simulink model "motor"  (R2015a)
settings: Solver=ode45  StartTime=0.0  StopTime=10.0  RelTol=1e-3
libraries: simulink x2
settings Model: Creator=joselo  LastModifiedBy=joselo

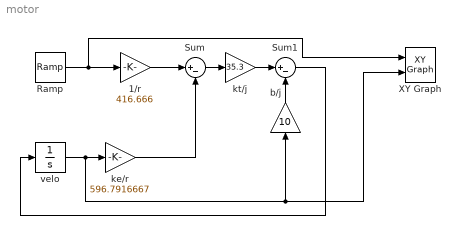
== system motor ==
  1/r : Gain  Gain=416.666
  Ramp : simulink/Sources/Ramp  slope=1  start=0  X0=0
  Sum : Sum  Inputs=|+-
  Sum1 : Sum  Inputs=|+-
  XY Graph : simulink/Sinks/XY Graph  xmin=-1  xmax=1  ymin=-1  ymax=1  st=-1
  b/j : Gain  Gain=10
  ke/r : Gain  Gain=596.7916667
  kt/j : Gain  Gain=35.3
  velo : Integrator
  wires:
  Ramp/1 -> XY Graph/1, 1/r/1
  1/r/1 -> Sum/1
  ke/r/1 -> Sum/2
  Sum/1 -> kt/j/1
  kt/j/1 -> Sum1/1
  b/j/1 -> Sum1/2
  velo/1 -> XY Graph/2, b/j/1, ke/r/1
  Sum1/1 -> velo/1
